simulink model "Five_Step_DTZNN"  (R2024a)
settings: Solver=ode4  StartTime=0.0  StopTime=10.0  FixedStep=0.01  RelTol=1e-3
values from neighbouring files (symbols this model uses):
  gamma = 1.0    (= 1)    [ctznn.m]    (also in setup.m = 40)
  tau = 0.01    [setup.m]
  X0 = rand(4,1)*2-1    [ctznn.m]    (also in setup.m = eye(2))
  X1 = X0 - tau*X0*dA(0)*X0 - h*X0*(A(0)*X0-eye(2))    [setup.m]
  X2 = X1 - tau*X1*dA(1*tau)*X1 - h*X1*(A(1*tau)*X1-eye(2))    [setup.m]
  X3 = X2 - tau*X2*dA(2*tau)*X2 - h*X2*(A(2*tau)*X2-eye(2))    [setup.m]
  X4 = X3 - tau*X3*dA(3*tau)*X3 - h*X3*(A(3*tau)*X3-eye(2))    [setup.m]
settings Model: Creator=uli_2  LastModifiedBy=uli_2
settings DebuggingCC: UnconnectedInputMsg=warning  UnconnectedOutputMsg=warning  UnconnectedLineMsg=warning
settings ModelReferenceCC: EnableRefExpFcnMdlSchedulingChecks=on
settings RTWCC: GPUComputeCapability=3.5  DLArmComputeVersion=19.05

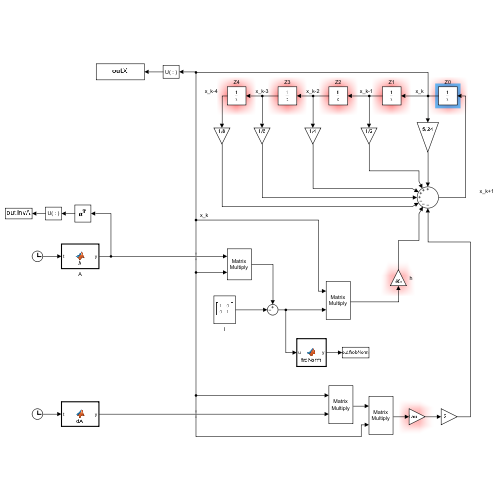
[thumbnail: Simulink's stored preview of the top-level diagram]
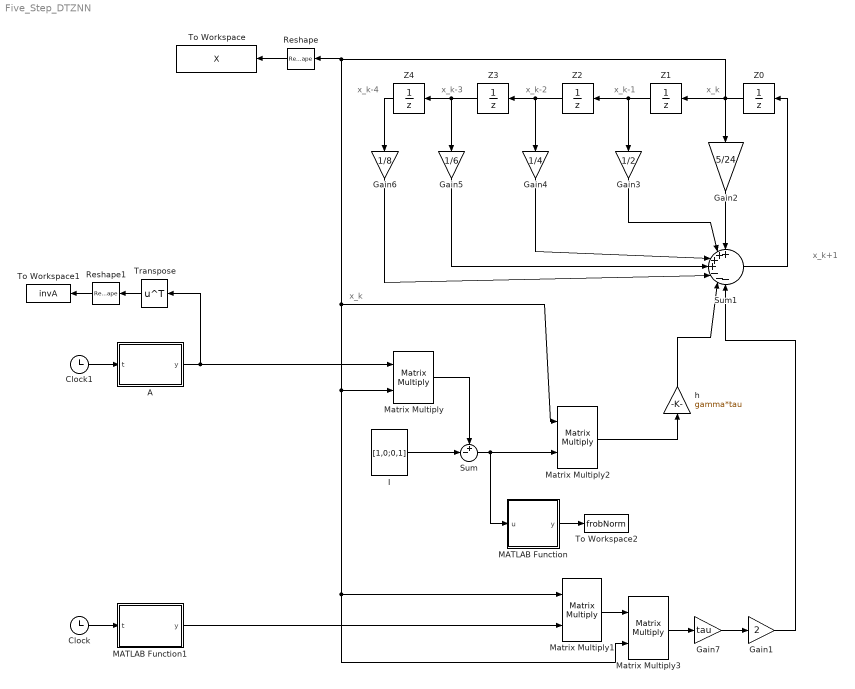
== system Five_Step_DTZNN ==
  note: x_k-3
  note: x_k-2
  note: x_k-1
  note: x_k
  note: x_k+1
  note: x_k
  note: x_k-4
  A : MATLAB Function  TreatAsAtomicUnit=on
  Clock : Clock
  Clock1 : Clock
  Gain1 : Gain  Gain=2
  Gain2 : Gain  Gain=5/24
  Gain3 : Gain  Gain=1/2
  Gain4 : Gain  Gain=1/4
  Gain5 : Gain  Gain=1/6
  Gain6 : Gain  Gain=1/8
  Gain7 : Gain  Gain=tau
  I : Constant  Value=[1,0;0,1]
  MATLAB Function : MATLAB Function  TreatAsAtomicUnit=on
  MATLAB Function1 : MATLAB Function  TreatAsAtomicUnit=on
  Matrix Multiply{,1..3} (4 alike) : Product  Multiplication=Matrix(*)
  Reshape : Reshape
  Reshape1 : Reshape
  Sum : Sum  Inputs=+-|
  Sum1 : Sum  Inputs=++++---
  To Workspace : ToWorkspace  VariableName=X  SaveFormat=Timeseries  SampleTime=-1
  To Workspace1 : ToWorkspace  VariableName=invA  SaveFormat=Timeseries  SampleTime=-1
  To Workspace2 : ToWorkspace  VariableName=frobNorm  SaveFormat=Timeseries  SampleTime=-1
  Transpose : Math  Operator=transpose
  Z0 : UnitDelay  InitialCondition=X4  SampleTime=-1  HasFrameUpgradeWarning=on
  Z1 : UnitDelay  InitialCondition=X3  SampleTime=-1  HasFrameUpgradeWarning=on
  Z2 : UnitDelay  InitialCondition=X2  SampleTime=-1  HasFrameUpgradeWarning=on
  Z3 : UnitDelay  InitialCondition=X1  SampleTime=-1  HasFrameUpgradeWarning=on
  Z4 : UnitDelay  InitialCondition=X0  SampleTime=-1  HasFrameUpgradeWarning=on
  h : Gain  Gain=gamma*tau
  wires:
  Z1/1 -> Z2/1, Gain3/1
  Sum1/1 -> Z0/1
  Matrix Multiply2/1 -> h/1
  Transpose/1 -> Reshape1/1
  Clock1/1 -> A/1(t)
  Clock/1 -> MATLAB Function1/1(t)
  Z2/1 -> Gain4/1, Z3/1
  Z3/1 -> Z4/1, Gain5/1
  Gain2/1 -> Sum1/1
  Gain3/1 -> Sum1/2
  Gain4/1 -> Sum1/3
  Gain5/1 -> Sum1/4
  Matrix Multiply/1 -> Sum/1
  Sum/1 -> MATLAB Function/1(u), Matrix Multiply2/2
  A/1(y) -> Matrix Multiply/1, Transpose/1
  I/1 -> Sum/2
  Z4/1 -> Gain6/1
  Gain6/1 -> Sum1/5
  h/1 -> Sum1/6
  MATLAB Function/1(y) -> To Workspace2/1
  MATLAB Function1/1(y) -> Matrix Multiply1/2
  Z0/1 -> Z1/1, Reshape/1, Matrix Multiply3/2, Matrix Multiply1/1, Matrix Multiply/2, Matrix Multiply2/1, Gain2/1
  Matrix Multiply1/1 -> Matrix Multiply3/1
  Matrix Multiply3/1 -> Gain7/1
  Gain7/1 -> Gain1/1
  Gain1/1 -> Sum1/7
  Reshape/1 -> To Workspace/1
  Reshape1/1 -> To Workspace1/1

== matlab function Five_Step_DTZNN/A ==
  data: t input; y output
function y = A(t)

y = [sin(t), cos(t); -cos(t), sin(t)];

== matlab function Five_Step_DTZNN/MATLAB Function ==
  data: u input; y output
function y = froNorm(u)
    y = norm(u, 'fro');

== matlab function Five_Step_DTZNN/MATLAB Function1 ==
  data: t input; y output
function y = dA(t)

y = [cos(t), -sin(t); sin(t), cos(t)];
